simulink model "LamBLHeatXEx"  (R2015a)
settings: Solver=FixedStepDiscrete  StartTime=0.0  StopTime=1500  FixedStep=dt  RelTol=1e-3
values from neighbouring files (symbols this model uses):
  Cp = 6.92*ones(length(y0),length(x))    [run_LamBLHeatXEx.m]
  k = 0.0328*ones(length(y0),length(x))    [run_LamBLHeatXEx.m]
  rho = 5.238864896*ones(length(y0),length(x))    [run_LamBLHeatXEx.m]
  rho_air = 0.00237    [run_LamBLHeatXEx.m]
  T0 = [T0; T0vec]    [run_LamBLHeatXEx.m]
  Te = 550    [run_LamBLHeatXEx.m]
  Uknown = 15    [run_LamBLHeatXEx.m]
  x = linspace(0,3,30)    [run_LamBLHeatXEx.m]
  xBL = linspace(0.05,3,50)    [run_LamBLHeatXEx.m]
  y = [y y0]    [run_LamBLHeatXEx.m]
libraries: lib_GenTools_1DlinearInterp x2, lib_AirProps_ThermCond x1, lib_AirProps_Viscosity x1, lib_Convection_FalknerSkanTempVary x1, lib_GenTools_PolynomialFit x1, lib_Conduction_2DCondFullyImplicit x1
settings Model: Creator=jlkratz  LastModifiedBy=jlkratz

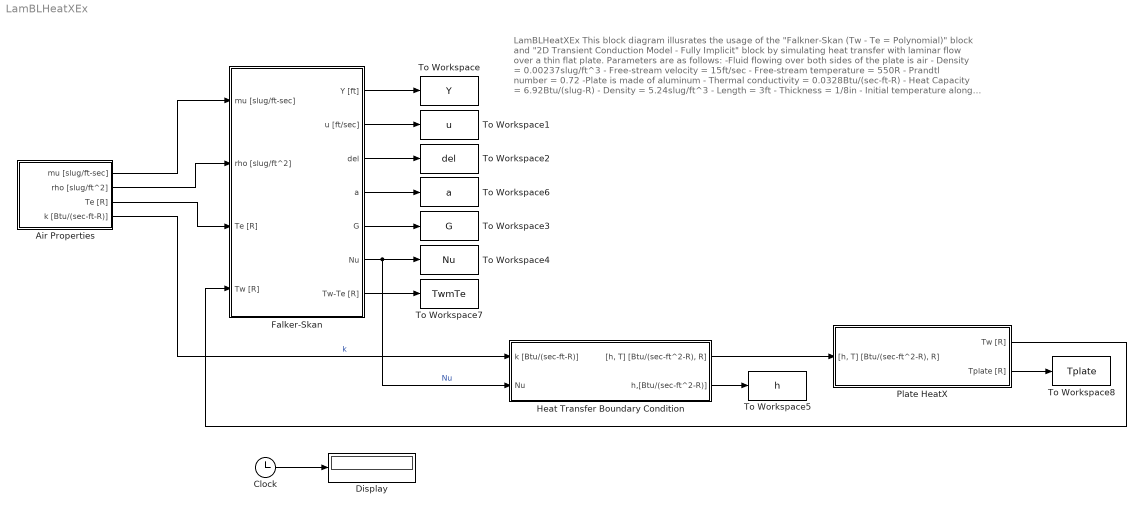
== system LamBLHeatXEx ==
  note: LamBLHeatXEx
      |
      | This block diagram illusrates the usage of the "Falkner-Skan (Tw - Te = Polynomial)" block and
      | "2D Transient Conduction Model - Fully Implicit" block by simulating heat transfer
      | with laminar flow over a thin flat plate. Parameters are as follows:
      | -Fluid flowing over both sides of the plate is air
      | - Density = 0.00237slug/ft^3
      | - Free-stream velocity = 15ft/sec
      | - Free-stream temperature = 550R
      | - Prandtl number = 0.72
      | -Plate is made of aluminum
      | - Thermal conductivity = 0.0328Btu/(sec-ft-R)
      | - Heat Capacity = 6.92Btu/(slug-R)
      | - Density = 5.24slug/ft^3
      | - Length = 3ft
      | - Thickness = 1/8in
      | - Initial temperature along the length follows the function: T0 = 800 - 20*x^2
  Air Properties : Subsystem
  Clock : Clock
  Display : Display
  Falker-Skan : Subsystem
  Heat Transfer Boundary Condition : Subsystem
  Plate HeatX : Subsystem
  To Workspace : ToWorkspace  VariableName=Y  SaveFormat=Timeseries  SampleTime=-1
  To Workspace1 : ToWorkspace  VariableName=u  SaveFormat=Timeseries  SampleTime=-1
  To Workspace2 : ToWorkspace  VariableName=del  SaveFormat=Timeseries  SampleTime=-1
  To Workspace3 : ToWorkspace  VariableName=G  SaveFormat=Timeseries  SampleTime=-1
  To Workspace4 : ToWorkspace  VariableName=Nu  SaveFormat=Timeseries  SampleTime=-1
  To Workspace5 : ToWorkspace  VariableName=h  SaveFormat=Timeseries  SampleTime=-1
  To Workspace6 : ToWorkspace  VariableName=a  SaveFormat=Timeseries  SampleTime=-1
  To Workspace7 : ToWorkspace  VariableName=TwmTe  SaveFormat=Timeseries  SampleTime=-1
  To Workspace8 : ToWorkspace  VariableName=Tplate  SaveFormat=Timeseries  SampleTime=-1
  wires:
  Falker-Skan/6(Nu) -> Heat Transfer Boundary Condition/2(Nu), To Workspace4/1  "Nu"
  Air Properties/1(mu [slug/ft-sec]) -> Falker-Skan/1(mu [slug/ft-sec])
  Air Properties/2(rho [slug/ft^2]) -> Falker-Skan/2(rho [slug/ft^2])
  Air Properties/3(Te [R]) -> Falker-Skan/3(Te [R])
  Falker-Skan/1(Y [ft]) -> To Workspace/1
  Falker-Skan/2(u [ft/sec]) -> To Workspace1/1
  Falker-Skan/3(del) -> To Workspace2/1
  Falker-Skan/4(a) -> To Workspace6/1
  Falker-Skan/5(G) -> To Workspace3/1
  Falker-Skan/7(Tw-Te [R]) -> To Workspace7/1
  Air Properties/4(k [Btu/(sec-ft-R)]) -> Heat Transfer Boundary Condition/1(k [Btu/(sec-ft-R)])  "k"
  Heat Transfer Boundary Condition/2(h,[Btu/(sec-ft^2-R)]) -> To Workspace5/1
  Heat Transfer Boundary Condition/1("[h, T] [Btu/(sec-ft^2-R), R]") -> Plate HeatX/1("[h, T] [Btu/(sec-ft^2-R), R]")
  Plate HeatX/1(Tw [R]) -> Falker-Skan/4(Tw [R])
  Plate HeatX/2(Tplate [R]) -> To Workspace8/1
  Clock/1 -> Display/1

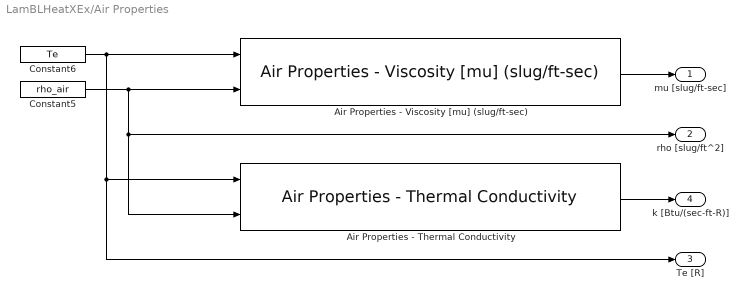
== system LamBLHeatXEx/Air Properties ==
  Air Properties - Thermal Conductivity : lib_AirProps_ThermCond/Air Properties - Thermal Conductivity  BN_M=double(gcb)
  Air Properties - Viscosity [mu] (slug/ft-sec) : lib_AirProps_Viscosity/Air Properties - Viscosity [mu] (slug//ft-sec)  BN_M=double(gcb)
  Constant5 : Constant  Value=rho_air
  Constant6 : Constant  Value=Te
  mu [slug/ft-sec] : Outport
  rho [slug/ft^2] : Outport  Port=2
  Te [R] : Outport  Port=3
  k [Btu/(sec-ft-R)] : Outport  Port=4
  wires:
  Air Properties - Thermal Conductivity/1 -> k [Btu/(sec-ft-R)]/1
  Constant5/1 -> Air Properties - Viscosity [mu] (slug/ft-sec)/2, rho [slug/ft^2]/1, Air Properties - Thermal Conductivity/2
  Constant6/1 -> Te [R]/1, Air Properties - Thermal Conductivity/1, Air Properties - Viscosity [mu] (slug/ft-sec)/1
  Air Properties - Viscosity [mu] (slug/ft-sec)/1 -> mu [slug/ft-sec]/1

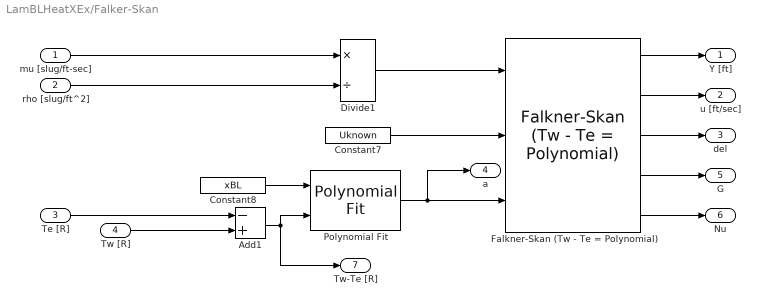
== system LamBLHeatXEx/Falker-Skan ==
  mu [slug/ft-sec] : Inport
  rho [slug/ft^2] : Inport  Port=2
  Te [R] : Inport  Port=3
  Tw [R] : Inport  Port=4
  Add1 : Sum  Inputs=-+
  Constant7 : Constant  Value=Uknown
  Constant8 : Constant  Value=xBL
  Divide1 : Product  Inputs=*/
  Falkner-Skan (Tw - Te = Polynomial) : lib_Convection_FalknerSkanTempVary/Falkner-Skan (Tw - Te = Polynomial)  Pr_M=Pr  beta_M=beta  x_Uknown_M=x_Uknown  x_M=xBL  n_M=n  imax_M=1000  BN_M=double(gcb)
  Polynomial Fit : lib_GenTools_PolynomialFit/Polynomial Fit  N_M=N  BN_M=double(gcb)
  Y [ft] : Outport
  u [ft/sec] : Outport  Port=2
  del : Outport  Port=3
  a : Outport  Port=4
  G : Outport  Port=5
  Nu : Outport  Port=6
  Tw-Te [R] : Outport  Port=7
  wires:
  mu [slug/ft-sec]/1 -> Divide1/1
  rho [slug/ft^2]/1 -> Divide1/2
  Te [R]/1 -> Add1/1
  Polynomial Fit/1 -> a/1, Falkner-Skan (Tw - Te = Polynomial)/3
  Falkner-Skan (Tw - Te = Polynomial)/1 -> Y [ft]/1
  Falkner-Skan (Tw - Te = Polynomial)/2 -> u [ft/sec]/1
  Falkner-Skan (Tw - Te = Polynomial)/3 -> del/1
  Falkner-Skan (Tw - Te = Polynomial)/4 -> G/1
  Falkner-Skan (Tw - Te = Polynomial)/5 -> Nu/1
  Divide1/1 -> Falkner-Skan (Tw - Te = Polynomial)/1
  Constant7/1 -> Falkner-Skan (Tw - Te = Polynomial)/2
  Constant8/1 -> Polynomial Fit/1
  Add1/1 -> Tw-Te [R]/1, Polynomial Fit/2
  Tw [R]/1 -> Add1/2

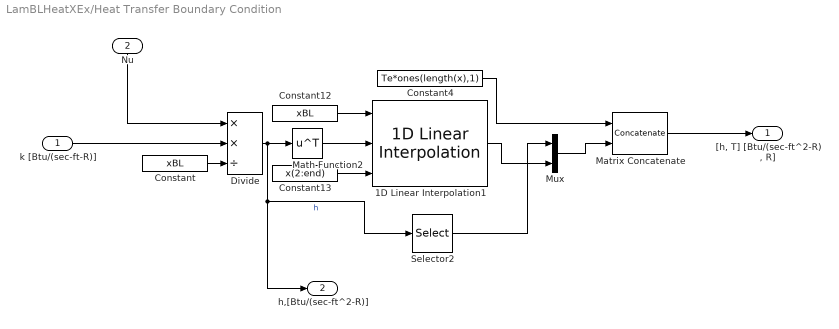
== system LamBLHeatXEx/Heat Transfer Boundary Condition ==
  k [Btu/(sec-ft-R)] : Inport
  Nu : Inport  Port=2
  1D Linear Interpolation1 : lib_GenTools_1DlinearInterp/1D Linear Interpolation  BN_M=double(gcb)
  Constant : Constant  Value=xBL
  Constant12 : Constant  Value=xBL
  Constant13 : Constant  Value=x(2:end)
  Constant4 : Constant  Value=Te*ones(length(x),1)
  Divide : Product  Inputs=**/
  Math Function2 : Math  Operator=transpose  SaturateOnIntegerOverflow=on
  Matrix Concatenate : Concatenate  Mode=Multidimensional array  ConcatenateDimension=2
  Mux : Mux  Inputs=2
  Selector2 : Selector  InputPortWidth=length(xBL)
  "[h, T] [Btu/(sec-ft^2-R), R]" : Outport
  h,[Btu/(sec-ft^2-R)] : Outport  Port=2
  wires:
  k [Btu/(sec-ft-R)]/1 -> Divide/2
  Mux/1 -> Matrix Concatenate/2
  Constant/1 -> Divide/3
  Matrix Concatenate/1 -> "[h, T] [Btu/(sec-ft^2-R), R]"/1
  Constant4/1 -> Matrix Concatenate/1
  Divide/1 -> Math Function2/1, h,[Btu/(sec-ft^2-R)]/1, Selector2/1  "h"
  Constant12/1 -> 1D Linear Interpolation1/1
  Constant13/1 -> 1D Linear Interpolation1/3
  1D Linear Interpolation1/1 -> Mux/2
  Selector2/1 -> Mux/1
  Nu/1 -> Divide/1
  Math Function2/1 -> 1D Linear Interpolation1/2

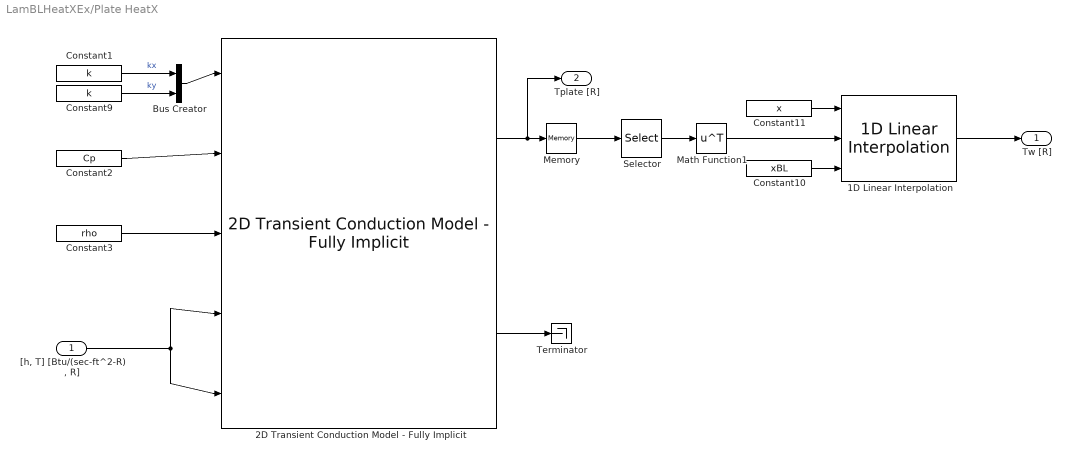
== system LamBLHeatXEx/Plate HeatX ==
  "[h, T] [Btu/(sec-ft^2-R), R]" : Inport
  1D Linear Interpolation : lib_GenTools_1DlinearInterp/1D Linear Interpolation  BN_M=double(gcb)
  2D Transient Conduction Model - Fully Implicit : lib_Conduction_2DCondFullyImplicit/2D Transient Conduction Model - Fully Implicit  T0_M=T0  dt_M=dt  x_M=x  y_M=y0  shape_M=Planar in both directions  convL_M=off  radL_M=off  condL_M=off  convR_M=off  radR_M=off  condR_M=off  convB_M=on  radB_M=off  condB_M=off  convT_M=on  radT_M=off  condT_M=off  BN_M=double(gcb)
  Bus Creator : BusCreator  Inputs=2
  Constant1 : Constant  Value=k
  Constant10 : Constant  Value=xBL
  Constant11 : Constant  Value=x
  Constant2 : Constant  Value=Cp
  Constant3 : Constant  Value=rho
  Constant9 : Constant  Value=k
  Math Function1 : Math  Operator=transpose  SaturateOnIntegerOverflow=on
  Memory : Memory  X0=T0
  Selector : Selector  NumberOfDimensions=2  InputPortWidth=3  IndexOptions=Index vector (dialog),Select all  Indices=size(y,1),1  OutputSizes=1,1
  Terminator : Terminator
  Tw [R] : Outport
  Tplate [R] : Outport  Port=2
  wires:
  2D Transient Conduction Model - Fully Implicit/1 -> Tplate [R]/1, Memory/1
  Constant3/1 -> 2D Transient Conduction Model - Fully Implicit/3
  Constant2/1 -> 2D Transient Conduction Model - Fully Implicit/2
  Memory/1 -> Selector/1
  Bus Creator/1 -> 2D Transient Conduction Model - Fully Implicit/1
  Constant1/1 -> Bus Creator/1  "kx"
  Constant9/1 -> Bus Creator/2  "ky"
  Constant10/1 -> 1D Linear Interpolation/3
  Constant11/1 -> 1D Linear Interpolation/1
  Selector/1 -> Math Function1/1
  "[h, T] [Btu/(sec-ft^2-R), R]"/1 -> 2D Transient Conduction Model - Fully Implicit/5, 2D Transient Conduction Model - Fully Implicit/4
  Math Function1/1 -> 1D Linear Interpolation/2
  1D Linear Interpolation/1 -> Tw [R]/1
  2D Transient Conduction Model - Fully Implicit/2 -> Terminator/1
